simulink model "blockdiagram"  (R2020a)
settings: Solver=ode4  StartTime=0.0  StopTime=12  FixedStep=0.001  RelTol=1e-3
values from neighbouring files (symbols this model uses):
  B = 0.05    [ProblemA.m]
  J = 0.1    [ProblemA.m]
  L2 = (Lmax-Lmin)/2    (= 0.04)    [ProblemA.m]
  theta_m0 = 0    [ProblemA.m]
undefined symbols (not defined in the file or in its folder): sigbuilder_block
libraries: simulink x6
(part 2 of 2)

== system blockdiagram/If Action Subsystem3/If Action Subsystem3 ==
  In1 : Inport
  Action Port : ActionPort  InitializeStates=reset  ActionPortLabel=if(u1 <-ep)
  Out1 : Outport
  wires:
  In1/1 -> Out1/1

== system blockdiagram/If Action Subsystem4/If Action Subsystem1 ==
  In1 : Inport
  Action Port : ActionPort  ActionPortLabel=else
  Constant14 : Constant  Value=-2*pi
  Mod13 : Math  Operator=mod  SaturateOnIntegerOverflow=on
  Out1 : Outport
  wires:
  In1/1 -> Mod13/1
  Constant14/1 -> Mod13/2
  Mod13/1 -> Out1/1

== system blockdiagram/If Action Subsystem4/If Action Subsystem3 ==
  In1 : Inport
  Action Port : ActionPort  InitializeStates=reset  ActionPortLabel=if(u1 <-ep)
  Out1 : Outport
  wires:
  In1/1 -> Out1/1

== system blockdiagram/If Action Subsystem5/Subsystem7 ==
  In1 : Inport
  Derivative1 : Derivative
  If Action Subsystem1 : Subsystem  TreatAsAtomicUnit=on
  If Action Subsystem3 : Subsystem  TreatAsAtomicUnit=on
  If2 : If  IfExpression=u1 < 0
  Merge2 : Merge
  Out1 : Outport
  wires:
  Derivative1/1 -> If2/1
  If2/2 -> If Action Subsystem1/Action
  If Action Subsystem1/1(Out1) -> Merge2/2
  If Action Subsystem3/1(Out2) -> Merge2/1
  If2/1 -> If Action Subsystem3/Action
  In1/1 -> If Action Subsystem3/1(In2), If Action Subsystem1/1(In1), Derivative1/1
  Merge2/1 -> Out1/1

== system blockdiagram/If Action Subsystem7/If Action Subsystem1 ==
  In1 : Inport
  Action Port : ActionPort  ActionPortLabel=if(u1<1.772)
  Subsystem7 : Subsystem
  Out1 : Outport
  wires:
  In1/1 -> Subsystem7/1(In1)
  Subsystem7/1(Out1) -> Out1/1

== system blockdiagram/If Action Subsystem7/If Action Subsystem7 ==
  In1 : Inport
  Action Port : ActionPort  ActionPortLabel=else
  Clock1 : Clock
  If Action Subsystem1 : Subsystem  TreatAsAtomicUnit=on
  If Action Subsystem7 : Subsystem  TreatAsAtomicUnit=on
  If4 : If  IfExpression=u1>9.658
  Merge2 : Merge
  Subsystem7 : Subsystem
  Out1 : Outport
  wires:
  Merge2/1 -> Out1/1
  If Action Subsystem7/1(Out1) -> Merge2/2
  In1/1 -> If Action Subsystem7/1(In1), If Action Subsystem1/1(In1)
  If4/2 -> If Action Subsystem7/Action
  Clock1/1 -> If4/1
  If4/1 -> If Action Subsystem1/Action
  If Action Subsystem1/1(Out1) -> Merge2/1

== system blockdiagram/If Action Subsystem7/Subsystem7 ==
  In1 : Inport
  Derivative1 : Derivative
  If Action Subsystem1 : Subsystem  TreatAsAtomicUnit=on
  If Action Subsystem3 : Subsystem  TreatAsAtomicUnit=on
  If2 : If  IfExpression=u1 < 0
  Merge2 : Merge
  Out1 : Outport
  wires:
  Derivative1/1 -> If2/1
  If2/2 -> If Action Subsystem1/Action
  If Action Subsystem1/1(Out1) -> Merge2/2
  If Action Subsystem3/1(Out2) -> Merge2/1
  If2/1 -> If Action Subsystem3/Action
  In1/1 -> If Action Subsystem3/1(In2), If Action Subsystem1/1(In1), Derivative1/1
  Merge2/1 -> Out1/1

== system blockdiagram/Subsystem/If Action Subsystem1 ==
  In1 : Inport
  Action Port : ActionPort  ActionPortLabel=else
  If Action Subsystem2 : Subsystem  TreatAsAtomicUnit=on
  If Action Subsystem4 : Subsystem  TreatAsAtomicUnit=on
  If1 : If  IfExpression=u1 <ep
  Merge1 : Merge
  Out1 : Outport
  wires:
  If1/1 -> If Action Subsystem4/Action
  If1/2 -> If Action Subsystem2/Action
  Merge1/1 -> Out1/1
  If Action Subsystem4/1(Out1) -> Merge1/1
  If Action Subsystem2/1(Out1) -> Merge1/2
  In1/1 -> If Action Subsystem2/1(In1), If Action Subsystem4/1(In1), If1/1

== system blockdiagram/Subsystem/If Action Subsystem3 ==
  In2 : Inport
  Action Port : ActionPort  InitializeStates=reset  ActionPortLabel=if(u1 < 0)
  Add : Sum  Inputs=+-
  Constant : Constant  Value=2*pi
  Constant14 : Constant  Value=-2*pi
  If Action Subsystem1 : Subsystem  TreatAsAtomicUnit=on
  If Action Subsystem3 : Subsystem  TreatAsAtomicUnit=on
  If2 : If  IfExpression=u1 <-ep
  Merge2 : Merge
  Mod13 : Math  Operator=mod  SaturateOnIntegerOverflow=on
  Out2 : Outport
  wires:
  Mod13/1 -> ?
  Constant14/1 -> Mod13/2
  ? -> Mod13/1
  Constant/1 -> Add/2
  In2/1 -> If Action Subsystem1/1(In1), If Action Subsystem3/1(In1), If2/1
  If Action Subsystem3/1(Out1) -> Merge2/1
  If2/1 -> If Action Subsystem3/Action
  If Action Subsystem1/1(Out1) -> Merge2/2
  If2/2 -> If Action Subsystem1/Action
  Merge2/1 -> Out2/1

== system blockdiagram/Subsystem1/If Action Subsystem1 ==
  In1 : Inport
  Action Port : ActionPort  ActionPortLabel=else
  Constant14 : Constant  Value=2*pi
  Mod13 : Math  Operator=mod  SaturateOnIntegerOverflow=on
  Out1 : Outport
  wires:
  In1/1 -> Mod13/1
  Constant14/1 -> Mod13/2
  Mod13/1 -> Out1/1

== system blockdiagram/Subsystem1/If Action Subsystem3 ==
  In1 : Inport
  Action Port : ActionPort  InitializeStates=reset  ActionPortLabel=if(u1 <ep)
  Out1 : Outport
  wires:
  In1/1 -> Out1/1

== system blockdiagram/Subsystem2/If Action Subsystem1 ==
  In1 : Inport
  Action Port : ActionPort  ActionPortLabel=else
  Constant14 : Constant  Value=2*pi
  Mod13 : Math  Operator=mod  SaturateOnIntegerOverflow=on
  Out1 : Outport
  wires:
  In1/1 -> Mod13/1
  Constant14/1 -> Mod13/2
  Mod13/1 -> Out1/1

== system blockdiagram/Subsystem2/If Action Subsystem3 ==
  In1 : Inport
  Action Port : ActionPort  InitializeStates=reset  ActionPortLabel=if(u1 <ep)
  Out1 : Outport
  wires:
  In1/1 -> Out1/1

== system blockdiagram/Subsystem3/If Action Subsystem1 ==
  In1 : Inport
  Action Port : ActionPort  ActionPortLabel=else
  Constant14 : Constant  Value=-2*pi
  Mod13 : Math  Operator=mod  SaturateOnIntegerOverflow=on
  Out1 : Outport
  wires:
  In1/1 -> Mod13/1
  Constant14/1 -> Mod13/2
  Mod13/1 -> Out1/1

== system blockdiagram/Subsystem3/If Action Subsystem3 ==
  In1 : Inport
  Action Port : ActionPort  InitializeStates=reset  ActionPortLabel=if(u1 <-ep)
  Out1 : Outport
  wires:
  In1/1 -> Out1/1

== system blockdiagram/Subsystem4/If Action Subsystem1 ==
  In1 : Inport
  Action Port : ActionPort  ActionPortLabel=else
  Constant14 : Constant  Value=-2*pi
  Mod13 : Math  Operator=mod  SaturateOnIntegerOverflow=on
  Out1 : Outport
  wires:
  In1/1 -> Mod13/1
  Constant14/1 -> Mod13/2
  Mod13/1 -> Out1/1

== system blockdiagram/Subsystem4/If Action Subsystem3 ==
  In1 : Inport
  Action Port : ActionPort  InitializeStates=reset  ActionPortLabel=if(u1 >-ep)
  Out1 : Outport
  wires:
  In1/1 -> Out1/1

== system blockdiagram/Subsystem5/If Action Subsystem1 ==
  In1 : Inport
  Action Port : ActionPort  ActionPortLabel=else
  If Action Subsystem2 : Subsystem  TreatAsAtomicUnit=on
  If Action Subsystem4 : Subsystem  TreatAsAtomicUnit=on
  If1 : If  IfExpression=u1 <ep
  Merge1 : Merge
  Out1 : Outport
  wires:
  If1/1 -> If Action Subsystem4/Action
  If1/2 -> If Action Subsystem2/Action
  Merge1/1 -> Out1/1
  If Action Subsystem4/1(Out1) -> Merge1/1
  If Action Subsystem2/1(Out1) -> Merge1/2
  In1/1 -> If Action Subsystem2/1(In1), If Action Subsystem4/1(In1), If1/1

== system blockdiagram/Subsystem5/If Action Subsystem3 ==
  In2 : Inport
  Action Port : ActionPort  InitializeStates=reset  ActionPortLabel=if(u1 < 0)
  Add : Sum  Inputs=+-
  Constant : Constant  Value=2*pi
  Constant14 : Constant  Value=-2*pi
  If Action Subsystem1 : Subsystem  TreatAsAtomicUnit=on
  If Action Subsystem3 : Subsystem  TreatAsAtomicUnit=on
  If2 : If  IfExpression=u1 <-ep
  Merge2 : Merge
  Mod13 : Math  Operator=mod  SaturateOnIntegerOverflow=on
  Out2 : Outport
  wires:
  Mod13/1 -> ?
  Constant14/1 -> Mod13/2
  ? -> Mod13/1
  Constant/1 -> Add/2
  In2/1 -> If Action Subsystem1/1(In1), If Action Subsystem3/1(In1), If2/1
  If Action Subsystem3/1(Out1) -> Merge2/1
  If2/1 -> If Action Subsystem3/Action
  If Action Subsystem1/1(Out1) -> Merge2/2
  If2/2 -> If Action Subsystem1/Action
  Merge2/1 -> Out2/1

== system blockdiagram/Subsystem6/If Action Subsystem1 ==
  In1 : Inport
  Action Port : ActionPort  ActionPortLabel=else
  If Action Subsystem2 : Subsystem  TreatAsAtomicUnit=on
  If Action Subsystem4 : Subsystem  TreatAsAtomicUnit=on
  If1 : If  IfExpression=u1 <ep
  Merge1 : Merge
  Out1 : Outport
  wires:
  If1/1 -> If Action Subsystem4/Action
  If1/2 -> If Action Subsystem2/Action
  Merge1/1 -> Out1/1
  If Action Subsystem4/1(Out1) -> Merge1/1
  If Action Subsystem2/1(Out1) -> Merge1/2
  In1/1 -> If Action Subsystem2/1(In1), If Action Subsystem4/1(In1), If1/1

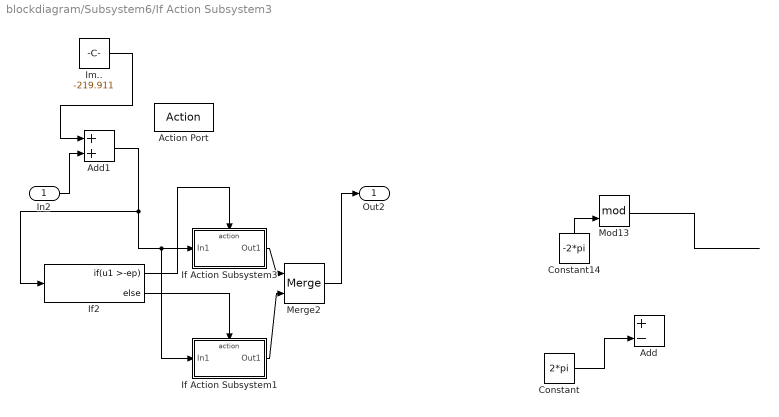
== system blockdiagram/Subsystem6/If Action Subsystem3 ==
  In2 : Inport
  Action Port : ActionPort  InitializeStates=reset  ActionPortLabel=if(u1 < 0)
  Add : Sum  Inputs=+-
  Add1 : Sum
  Constant : Constant  Value=2*pi
  Constant14 : Constant  Value=-2*pi
  If Action Subsystem1 : Subsystem  TreatAsAtomicUnit=on
  If Action Subsystem3 : Subsystem  TreatAsAtomicUnit=on
  If2 : If  IfExpression=u1 >-ep
  Im.. : Constant  Value=-219.911
  Merge2 : Merge
  Mod13 : Math  Operator=mod  SaturateOnIntegerOverflow=on
  Out2 : Outport
  wires:
  Mod13/1 -> ?
  Constant14/1 -> Mod13/2
  ? -> Mod13/1
  Constant/1 -> Add/2
  If Action Subsystem3/1(Out1) -> Merge2/1
  If2/1 -> If Action Subsystem3/Action
  If Action Subsystem1/1(Out1) -> Merge2/2
  If2/2 -> If Action Subsystem1/Action
  Merge2/1 -> Out2/1
  Im../1 -> Add1/1
  In2/1 -> Add1/2
  Add1/1 -> If Action Subsystem3/1(In1), If Action Subsystem1/1(In1), If2/1

== system blockdiagram/Subsystem7/If Action Subsystem1 ==
  In1 : Inport
  Action Port : ActionPort  ActionPortLabel=else
  If Action Subsystem2 : Subsystem  TreatAsAtomicUnit=on
  If Action Subsystem4 : Subsystem  TreatAsAtomicUnit=on
  If1 : If  IfExpression=u1 <ep
  Merge1 : Merge
  Out1 : Outport
  wires:
  If1/1 -> If Action Subsystem4/Action
  If1/2 -> If Action Subsystem2/Action
  Merge1/1 -> Out1/1
  If Action Subsystem4/1(Out1) -> Merge1/1
  If Action Subsystem2/1(Out1) -> Merge1/2
  In1/1 -> If Action Subsystem2/1(In1), If Action Subsystem4/1(In1), If1/1

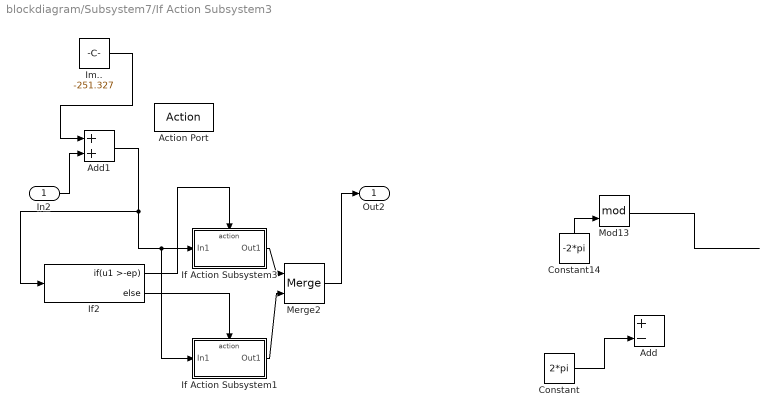
== system blockdiagram/Subsystem7/If Action Subsystem3 ==
  In2 : Inport
  Action Port : ActionPort  InitializeStates=reset  ActionPortLabel=if(u1 < 0)
  Add : Sum  Inputs=+-
  Add1 : Sum
  Constant : Constant  Value=2*pi
  Constant14 : Constant  Value=-2*pi
  If Action Subsystem1 : Subsystem  TreatAsAtomicUnit=on
  If Action Subsystem3 : Subsystem  TreatAsAtomicUnit=on
  If2 : If  IfExpression=u1 >-ep
  Im.. : Constant  Value=-251.327
  Merge2 : Merge
  Mod13 : Math  Operator=mod  SaturateOnIntegerOverflow=on
  Out2 : Outport
  wires:
  Mod13/1 -> ?
  Constant14/1 -> Mod13/2
  ? -> Mod13/1
  Constant/1 -> Add/2
  If Action Subsystem3/1(Out1) -> Merge2/1
  If2/1 -> If Action Subsystem3/Action
  If Action Subsystem1/1(Out1) -> Merge2/2
  If2/2 -> If Action Subsystem1/Action
  Merge2/1 -> Out2/1
  Im../1 -> Add1/1
  In2/1 -> Add1/2
  Add1/1 -> If Action Subsystem3/1(In1), If Action Subsystem1/1(In1), If2/1

== system blockdiagram/Subsystem8/If Action Subsystem1 ==
  In1 : Inport
  Action Port : ActionPort  ActionPortLabel=else
  If Action Subsystem2 : Subsystem  TreatAsAtomicUnit=on
  If Action Subsystem4 : Subsystem  TreatAsAtomicUnit=on
  If1 : If  IfExpression=u1 <ep
  Merge1 : Merge
  Out1 : Outport
  wires:
  If1/1 -> If Action Subsystem4/Action
  If1/2 -> If Action Subsystem2/Action
  Merge1/1 -> Out1/1
  If Action Subsystem4/1(Out1) -> Merge1/1
  If Action Subsystem2/1(Out1) -> Merge1/2
  In1/1 -> If Action Subsystem2/1(In1), If Action Subsystem4/1(In1), If1/1

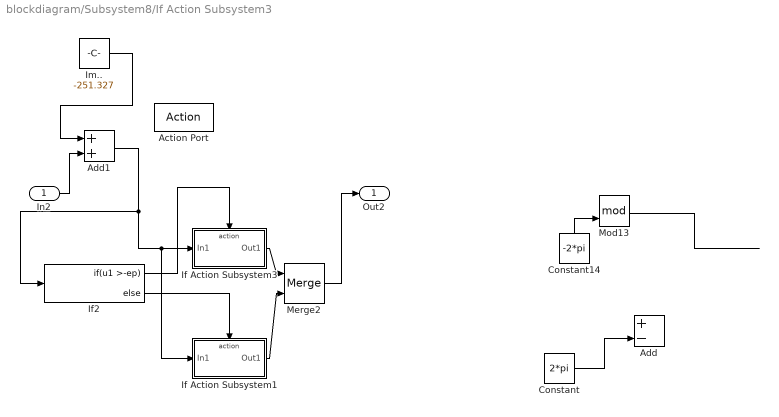
== system blockdiagram/Subsystem8/If Action Subsystem3 ==
  In2 : Inport
  Action Port : ActionPort  InitializeStates=reset  ActionPortLabel=if(u1 < 0)
  Add : Sum  Inputs=+-
  Add1 : Sum
  Constant : Constant  Value=2*pi
  Constant14 : Constant  Value=-2*pi
  If Action Subsystem1 : Subsystem  TreatAsAtomicUnit=on
  If Action Subsystem3 : Subsystem  TreatAsAtomicUnit=on
  If2 : If  IfExpression=u1 >-ep
  Im.. : Constant  Value=-251.327
  Merge2 : Merge
  Mod13 : Math  Operator=mod  SaturateOnIntegerOverflow=on
  Out2 : Outport
  wires:
  Mod13/1 -> ?
  Constant14/1 -> Mod13/2
  ? -> Mod13/1
  Constant/1 -> Add/2
  If Action Subsystem3/1(Out1) -> Merge2/1
  If2/1 -> If Action Subsystem3/Action
  If Action Subsystem1/1(Out1) -> Merge2/2
  If2/2 -> If Action Subsystem1/Action
  Merge2/1 -> Out2/1
  Im../1 -> Add1/1
  In2/1 -> Add1/2
  Add1/1 -> If Action Subsystem3/1(In1), If Action Subsystem1/1(In1), If2/1

== system blockdiagram/If Action Subsystem5/Subsystem7/If Action Subsystem1 ==
  In1 : Inport
  Action Port : ActionPort  ActionPortLabel=else
  If Action Subsystem2 : Subsystem  TreatAsAtomicUnit=on
  If Action Subsystem4 : Subsystem  TreatAsAtomicUnit=on
  If1 : If  IfExpression=u1 <ep
  Merge1 : Merge
  Out1 : Outport
  wires:
  If1/1 -> If Action Subsystem4/Action
  If1/2 -> If Action Subsystem2/Action
  Merge1/1 -> Out1/1
  If Action Subsystem4/1(Out1) -> Merge1/1
  If Action Subsystem2/1(Out1) -> Merge1/2
  In1/1 -> If Action Subsystem2/1(In1), If Action Subsystem4/1(In1), If1/1

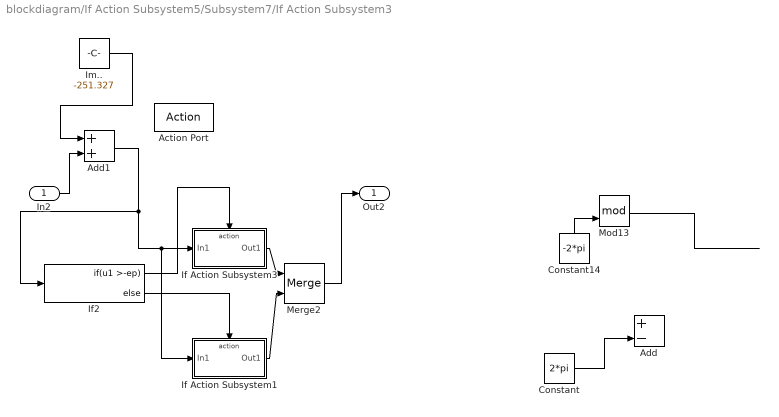
== system blockdiagram/If Action Subsystem5/Subsystem7/If Action Subsystem3 ==
  In2 : Inport
  Action Port : ActionPort  InitializeStates=reset  ActionPortLabel=if(u1 < 0)
  Add : Sum  Inputs=+-
  Add1 : Sum
  Constant : Constant  Value=2*pi
  Constant14 : Constant  Value=-2*pi
  If Action Subsystem1 : Subsystem  TreatAsAtomicUnit=on
  If Action Subsystem3 : Subsystem  TreatAsAtomicUnit=on
  If2 : If  IfExpression=u1 >-ep
  Im.. : Constant  Value=-251.327
  Merge2 : Merge
  Mod13 : Math  Operator=mod  SaturateOnIntegerOverflow=on
  Out2 : Outport
  wires:
  Mod13/1 -> ?
  Constant14/1 -> Mod13/2
  ? -> Mod13/1
  Constant/1 -> Add/2
  If Action Subsystem3/1(Out1) -> Merge2/1
  If2/1 -> If Action Subsystem3/Action
  If Action Subsystem1/1(Out1) -> Merge2/2
  If2/2 -> If Action Subsystem1/Action
  Merge2/1 -> Out2/1
  Im../1 -> Add1/1
  In2/1 -> Add1/2
  Add1/1 -> If Action Subsystem3/1(In1), If Action Subsystem1/1(In1), If2/1

== system blockdiagram/If Action Subsystem7/If Action Subsystem1/Subsystem7 ==
  In1 : Inport
  Derivative1 : Derivative
  If Action Subsystem1 : Subsystem  TreatAsAtomicUnit=on
  If Action Subsystem3 : Subsystem  TreatAsAtomicUnit=on
  If2 : If  IfExpression=u1 < 0
  Merge2 : Merge
  Out1 : Outport
  wires:
  Derivative1/1 -> If2/1
  If2/2 -> If Action Subsystem1/Action
  If Action Subsystem1/1(Out1) -> Merge2/2
  If Action Subsystem3/1(Out2) -> Merge2/1
  If2/1 -> If Action Subsystem3/Action
  In1/1 -> If Action Subsystem3/1(In2), If Action Subsystem1/1(In1), Derivative1/1
  Merge2/1 -> Out1/1

== system blockdiagram/If Action Subsystem7/If Action Subsystem7/If Action Subsystem1 ==
  In1 : Inport
  Action Port : ActionPort  ActionPortLabel=if(u1>9.658)
  Subsystem7 : Subsystem
  Out1 : Outport
  wires:
  In1/1 -> Subsystem7/1(In1)
  Subsystem7/1(Out1) -> Out1/1

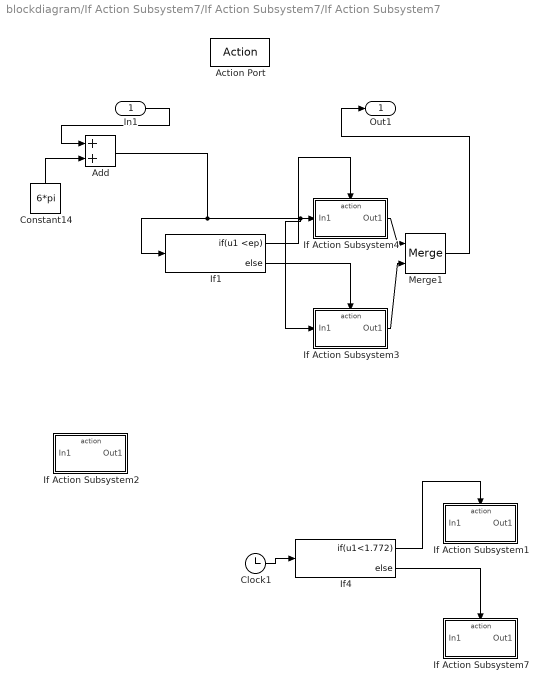
== system blockdiagram/If Action Subsystem7/If Action Subsystem7/If Action Subsystem7 ==
  In1 : Inport
  Action Port : ActionPort  ActionPortLabel=else
  Add : Sum
  Clock1 : Clock
  Constant14 : Constant  Value=6*pi
  If Action Subsystem1 : Subsystem  TreatAsAtomicUnit=on
  If Action Subsystem2 : Subsystem  TreatAsAtomicUnit=on
  If Action Subsystem3 : Subsystem  TreatAsAtomicUnit=on
  If Action Subsystem4 : Subsystem  TreatAsAtomicUnit=on
  If Action Subsystem7 : Subsystem  TreatAsAtomicUnit=on
  If1 : If  IfExpression=u1 <ep
  If4 : If  IfExpression=u1<1.772
  Merge1 : Merge
  Out1 : Outport
  wires:
  Merge1/1 -> Out1/1
  If4/2 -> If Action Subsystem7/Action
  Clock1/1 -> If4/1
  ? -> If Action Subsystem1/1(In1), If Action Subsystem7/1(In1)
  If4/1 -> If Action Subsystem1/Action
  If1/1 -> If Action Subsystem4/Action
  If Action Subsystem4/1(Out1) -> Merge1/1
  If1/2 -> If Action Subsystem3/Action
  If Action Subsystem3/1(Out1) -> Merge1/2
  Add/1 -> If1/1, If Action Subsystem3/1(In1), If Action Subsystem4/1(In1)
  In1/1 -> Add/1
  Constant14/1 -> Add/2

== system blockdiagram/If Action Subsystem7/If Action Subsystem7/Subsystem7 ==
  In1 : Inport
  Derivative1 : Derivative
  If Action Subsystem1 : Subsystem  TreatAsAtomicUnit=on
  If Action Subsystem3 : Subsystem  TreatAsAtomicUnit=on
  If2 : If  IfExpression=u1 < 0
  Merge2 : Merge
  Out1 : Outport
  wires:
  Derivative1/1 -> If2/1
  If2/2 -> If Action Subsystem1/Action
  If Action Subsystem1/1(Out1) -> Merge2/2
  If Action Subsystem3/1(Out2) -> Merge2/1
  If2/1 -> If Action Subsystem3/Action
  In1/1 -> If Action Subsystem3/1(In2), If Action Subsystem1/1(In1), Derivative1/1
  Merge2/1 -> Out1/1

== system blockdiagram/If Action Subsystem7/Subsystem7/If Action Subsystem1 ==
  In1 : Inport
  Action Port : ActionPort  ActionPortLabel=else
  If Action Subsystem2 : Subsystem  TreatAsAtomicUnit=on
  If Action Subsystem4 : Subsystem  TreatAsAtomicUnit=on
  If1 : If  IfExpression=u1 <ep
  Merge1 : Merge
  Out1 : Outport
  wires:
  If1/1 -> If Action Subsystem4/Action
  If1/2 -> If Action Subsystem2/Action
  Merge1/1 -> Out1/1
  If Action Subsystem4/1(Out1) -> Merge1/1
  If Action Subsystem2/1(Out1) -> Merge1/2
  In1/1 -> If Action Subsystem2/1(In1), If Action Subsystem4/1(In1), If1/1

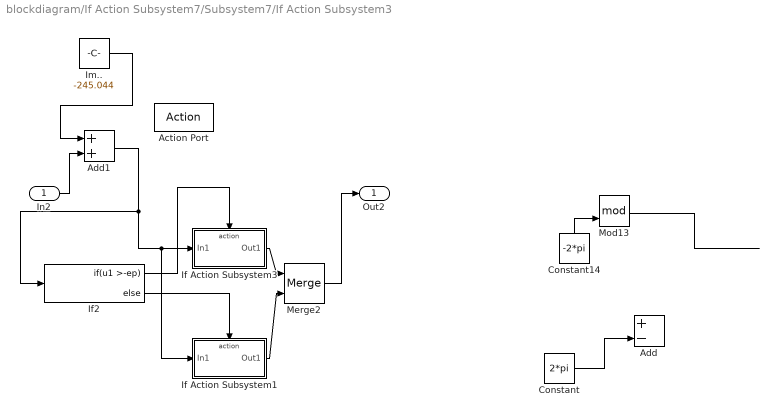
== system blockdiagram/If Action Subsystem7/Subsystem7/If Action Subsystem3 ==
  In2 : Inport
  Action Port : ActionPort  InitializeStates=reset  ActionPortLabel=if(u1 < 0)
  Add : Sum  Inputs=+-
  Add1 : Sum
  Constant : Constant  Value=2*pi
  Constant14 : Constant  Value=-2*pi
  If Action Subsystem1 : Subsystem  TreatAsAtomicUnit=on
  If Action Subsystem3 : Subsystem  TreatAsAtomicUnit=on
  If2 : If  IfExpression=u1 >-ep
  Im.. : Constant  Value=-245.044
  Merge2 : Merge
  Mod13 : Math  Operator=mod  SaturateOnIntegerOverflow=on
  Out2 : Outport
  wires:
  Mod13/1 -> ?
  Constant14/1 -> Mod13/2
  ? -> Mod13/1
  Constant/1 -> Add/2
  If Action Subsystem3/1(Out1) -> Merge2/1
  If2/1 -> If Action Subsystem3/Action
  If Action Subsystem1/1(Out1) -> Merge2/2
  If2/2 -> If Action Subsystem1/Action
  Merge2/1 -> Out2/1
  Im../1 -> Add1/1
  In2/1 -> Add1/2
  Add1/1 -> If Action Subsystem3/1(In1), If Action Subsystem1/1(In1), If2/1

== system blockdiagram/Subsystem/If Action Subsystem1/If Action Subsystem2 ==
  In1 : Inport
  Action Port : ActionPort  ActionPortLabel=else
  Constant14 : Constant  Value=2*pi
  Mod13 : Math  Operator=mod  SaturateOnIntegerOverflow=on
  Out1 : Outport
  wires:
  In1/1 -> Mod13/1
  Constant14/1 -> Mod13/2
  Mod13/1 -> Out1/1

== system blockdiagram/Subsystem/If Action Subsystem1/If Action Subsystem4 ==
  In1 : Inport
  Action Port : ActionPort  InitializeStates=reset  ActionPortLabel=if(u1 <ep)
  Out1 : Outport
  wires:
  In1/1 -> Out1/1

== system blockdiagram/Subsystem/If Action Subsystem3/If Action Subsystem1 ==
  In1 : Inport
  Action Port : ActionPort  ActionPortLabel=else
  Constant14 : Constant  Value=-2*pi
  Mod13 : Math  Operator=mod  SaturateOnIntegerOverflow=on
  Out1 : Outport
  wires:
  In1/1 -> Mod13/1
  Constant14/1 -> Mod13/2
  Mod13/1 -> Out1/1

== system blockdiagram/Subsystem/If Action Subsystem3/If Action Subsystem3 ==
  In1 : Inport
  Action Port : ActionPort  InitializeStates=reset  ActionPortLabel=if(u1 <-ep)
  Out1 : Outport
  wires:
  In1/1 -> Out1/1

== system blockdiagram/Subsystem5/If Action Subsystem1/If Action Subsystem2 ==
  In1 : Inport
  Action Port : ActionPort  ActionPortLabel=else
  Constant14 : Constant  Value=2*pi
  Mod13 : Math  Operator=mod  SaturateOnIntegerOverflow=on
  Out1 : Outport
  wires:
  In1/1 -> Mod13/1
  Constant14/1 -> Mod13/2
  Mod13/1 -> Out1/1

== system blockdiagram/Subsystem5/If Action Subsystem1/If Action Subsystem4 ==
  In1 : Inport
  Action Port : ActionPort  InitializeStates=reset  ActionPortLabel=if(u1 <ep)
  Out1 : Outport
  wires:
  In1/1 -> Out1/1

== system blockdiagram/Subsystem5/If Action Subsystem3/If Action Subsystem1 ==
  In1 : Inport
  Action Port : ActionPort  ActionPortLabel=else
  Constant14 : Constant  Value=-2*pi
  Mod13 : Math  Operator=mod  SaturateOnIntegerOverflow=on
  Out1 : Outport
  wires:
  In1/1 -> Mod13/1
  Constant14/1 -> Mod13/2
  Mod13/1 -> Out1/1

== system blockdiagram/Subsystem5/If Action Subsystem3/If Action Subsystem3 ==
  In1 : Inport
  Action Port : ActionPort  InitializeStates=reset  ActionPortLabel=if(u1 <-ep)
  Out1 : Outport
  wires:
  In1/1 -> Out1/1

== system blockdiagram/Subsystem6/If Action Subsystem1/If Action Subsystem2 ==
  In1 : Inport
  Action Port : ActionPort  ActionPortLabel=else
  Constant14 : Constant  Value=2*pi
  Mod13 : Math  Operator=mod  SaturateOnIntegerOverflow=on
  Out1 : Outport
  wires:
  In1/1 -> Mod13/1
  Constant14/1 -> Mod13/2
  Mod13/1 -> Out1/1

== system blockdiagram/Subsystem6/If Action Subsystem1/If Action Subsystem4 ==
  In1 : Inport
  Action Port : ActionPort  InitializeStates=reset  ActionPortLabel=if(u1 <ep)
  Out1 : Outport
  wires:
  In1/1 -> Out1/1

== system blockdiagram/Subsystem6/If Action Subsystem3/If Action Subsystem1 ==
  In1 : Inport
  Action Port : ActionPort  ActionPortLabel=else
  Constant14 : Constant  Value=-2*pi
  Mod13 : Math  Operator=mod  SaturateOnIntegerOverflow=on
  Out1 : Outport
  wires:
  In1/1 -> Mod13/1
  Constant14/1 -> Mod13/2
  Mod13/1 -> Out1/1

== system blockdiagram/Subsystem6/If Action Subsystem3/If Action Subsystem3 ==
  In1 : Inport
  Action Port : ActionPort  InitializeStates=reset  ActionPortLabel=if(u1 >-ep)
  Out1 : Outport
  wires:
  In1/1 -> Out1/1

== system blockdiagram/Subsystem7/If Action Subsystem1/If Action Subsystem2 ==
  In1 : Inport
  Action Port : ActionPort  ActionPortLabel=else
  Constant14 : Constant  Value=2*pi
  Mod13 : Math  Operator=mod  SaturateOnIntegerOverflow=on
  Out1 : Outport
  wires:
  In1/1 -> Mod13/1
  Constant14/1 -> Mod13/2
  Mod13/1 -> Out1/1

== system blockdiagram/Subsystem7/If Action Subsystem1/If Action Subsystem4 ==
  In1 : Inport
  Action Port : ActionPort  InitializeStates=reset  ActionPortLabel=if(u1 <ep)
  Out1 : Outport
  wires:
  In1/1 -> Out1/1

== system blockdiagram/Subsystem7/If Action Subsystem3/If Action Subsystem1 ==
  In1 : Inport
  Action Port : ActionPort  ActionPortLabel=else
  Constant14 : Constant  Value=-2*pi
  Mod13 : Math  Operator=mod  SaturateOnIntegerOverflow=on
  Out1 : Outport
  wires:
  In1/1 -> Mod13/1
  Constant14/1 -> Mod13/2
  Mod13/1 -> Out1/1

== system blockdiagram/Subsystem7/If Action Subsystem3/If Action Subsystem3 ==
  In1 : Inport
  Action Port : ActionPort  InitializeStates=reset  ActionPortLabel=if(u1 >-ep)
  Out1 : Outport
  wires:
  In1/1 -> Out1/1

== system blockdiagram/Subsystem8/If Action Subsystem1/If Action Subsystem2 ==
  In1 : Inport
  Action Port : ActionPort  ActionPortLabel=else
  Constant14 : Constant  Value=2*pi
  Mod13 : Math  Operator=mod  SaturateOnIntegerOverflow=on
  Out1 : Outport
  wires:
  In1/1 -> Mod13/1
  Constant14/1 -> Mod13/2
  Mod13/1 -> Out1/1

== system blockdiagram/Subsystem8/If Action Subsystem1/If Action Subsystem4 ==
  In1 : Inport
  Action Port : ActionPort  InitializeStates=reset  ActionPortLabel=if(u1 <ep)
  Out1 : Outport
  wires:
  In1/1 -> Out1/1

== system blockdiagram/Subsystem8/If Action Subsystem3/If Action Subsystem1 ==
  In1 : Inport
  Action Port : ActionPort  ActionPortLabel=else
  Constant14 : Constant  Value=-2*pi
  Mod13 : Math  Operator=mod  SaturateOnIntegerOverflow=on
  Out1 : Outport
  wires:
  In1/1 -> Mod13/1
  Constant14/1 -> Mod13/2
  Mod13/1 -> Out1/1

== system blockdiagram/Subsystem8/If Action Subsystem3/If Action Subsystem3 ==
  In1 : Inport
  Action Port : ActionPort  InitializeStates=reset  ActionPortLabel=if(u1 >-ep)
  Out1 : Outport
  wires:
  In1/1 -> Out1/1

== system blockdiagram/If Action Subsystem5/Subsystem7/If Action Subsystem1/If Action Subsystem2 ==
  In1 : Inport
  Action Port : ActionPort  ActionPortLabel=else
  Constant14 : Constant  Value=2*pi
  Mod13 : Math  Operator=mod  SaturateOnIntegerOverflow=on
  Out1 : Outport
  wires:
  In1/1 -> Mod13/1
  Constant14/1 -> Mod13/2
  Mod13/1 -> Out1/1

== system blockdiagram/If Action Subsystem5/Subsystem7/If Action Subsystem1/If Action Subsystem4 ==
  In1 : Inport
  Action Port : ActionPort  InitializeStates=reset  ActionPortLabel=if(u1 <ep)
  Out1 : Outport
  wires:
  In1/1 -> Out1/1

== system blockdiagram/If Action Subsystem5/Subsystem7/If Action Subsystem3/If Action Subsystem1 ==
  In1 : Inport
  Action Port : ActionPort  ActionPortLabel=else
  Constant14 : Constant  Value=-2*pi
  Mod13 : Math  Operator=mod  SaturateOnIntegerOverflow=on
  Out1 : Outport
  wires:
  In1/1 -> Mod13/1
  Constant14/1 -> Mod13/2
  Mod13/1 -> Out1/1

== system blockdiagram/If Action Subsystem5/Subsystem7/If Action Subsystem3/If Action Subsystem3 ==
  In1 : Inport
  Action Port : ActionPort  InitializeStates=reset  ActionPortLabel=if(u1 >-ep)
  Out1 : Outport
  wires:
  In1/1 -> Out1/1

== system blockdiagram/If Action Subsystem7/If Action Subsystem1/Subsystem7/If Action Subsystem1 ==
  In1 : Inport
  Action Port : ActionPort  ActionPortLabel=else
  If Action Subsystem2 : Subsystem  TreatAsAtomicUnit=on
  If Action Subsystem4 : Subsystem  TreatAsAtomicUnit=on
  If1 : If  IfExpression=u1 <ep
  Merge1 : Merge
  Out1 : Outport
  wires:
  If1/1 -> If Action Subsystem4/Action
  If1/2 -> If Action Subsystem2/Action
  Merge1/1 -> Out1/1
  If Action Subsystem4/1(Out1) -> Merge1/1
  If Action Subsystem2/1(Out1) -> Merge1/2
  In1/1 -> If Action Subsystem2/1(In1), If Action Subsystem4/1(In1), If1/1

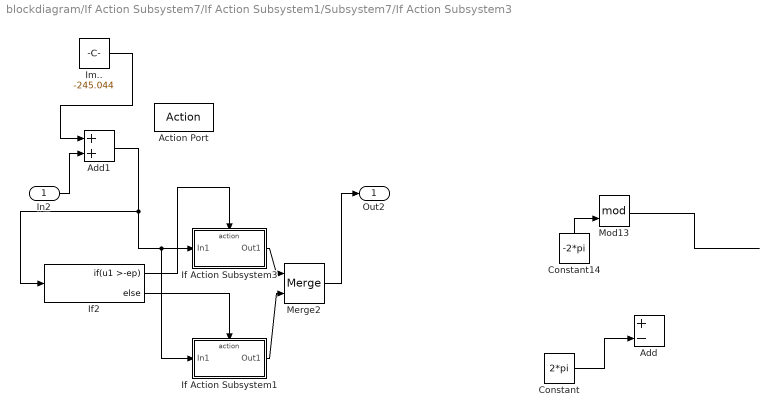
== system blockdiagram/If Action Subsystem7/If Action Subsystem1/Subsystem7/If Action Subsystem3 ==
  In2 : Inport
  Action Port : ActionPort  InitializeStates=reset  ActionPortLabel=if(u1 < 0)
  Add : Sum  Inputs=+-
  Add1 : Sum
  Constant : Constant  Value=2*pi
  Constant14 : Constant  Value=-2*pi
  If Action Subsystem1 : Subsystem  TreatAsAtomicUnit=on
  If Action Subsystem3 : Subsystem  TreatAsAtomicUnit=on
  If2 : If  IfExpression=u1 >-ep
  Im.. : Constant  Value=-245.044
  Merge2 : Merge
  Mod13 : Math  Operator=mod  SaturateOnIntegerOverflow=on
  Out2 : Outport
  wires:
  Mod13/1 -> ?
  Constant14/1 -> Mod13/2
  ? -> Mod13/1
  Constant/1 -> Add/2
  If Action Subsystem3/1(Out1) -> Merge2/1
  If2/1 -> If Action Subsystem3/Action
  If Action Subsystem1/1(Out1) -> Merge2/2
  If2/2 -> If Action Subsystem1/Action
  Merge2/1 -> Out2/1
  Im../1 -> Add1/1
  In2/1 -> Add1/2
  Add1/1 -> If Action Subsystem3/1(In1), If Action Subsystem1/1(In1), If2/1

== system blockdiagram/If Action Subsystem7/If Action Subsystem7/If Action Subsystem1/Subsystem7 ==
  In1 : Inport
  Derivative1 : Derivative
  If Action Subsystem1 : Subsystem  TreatAsAtomicUnit=on
  If Action Subsystem3 : Subsystem  TreatAsAtomicUnit=on
  If2 : If  IfExpression=u1 < 0
  Merge2 : Merge
  Out1 : Outport
  wires:
  Derivative1/1 -> If2/1
  If2/2 -> If Action Subsystem1/Action
  If Action Subsystem1/1(Out1) -> Merge2/2
  If Action Subsystem3/1(Out2) -> Merge2/1
  If2/1 -> If Action Subsystem3/Action
  In1/1 -> If Action Subsystem3/1(In2), If Action Subsystem1/1(In1), Derivative1/1
  Merge2/1 -> Out1/1

== system blockdiagram/If Action Subsystem7/If Action Subsystem7/If Action Subsystem7/If Action Subsystem1 ==
  In1 : Inport
  Action Port : ActionPort  ActionPortLabel=if(u1<1.772)
  Subsystem7 : Subsystem
  Out1 : Outport
  wires:
  In1/1 -> Subsystem7/1(In1)
  Subsystem7/1(Out1) -> Out1/1

== system blockdiagram/If Action Subsystem7/If Action Subsystem7/If Action Subsystem7/If Action Subsystem2 ==
  In1 : Inport
  Action Port : ActionPort
  If Action Subsystem2 : Subsystem  TreatAsAtomicUnit=on
  If Action Subsystem4 : Subsystem  TreatAsAtomicUnit=on
  If1 : If  IfExpression=u1 <ep
  Merge1 : Merge
  Out1 : Outport
  wires:
  If1/1 -> If Action Subsystem4/Action
  If1/2 -> If Action Subsystem2/Action
  Merge1/1 -> Out1/1
  If Action Subsystem4/1(Out1) -> Merge1/1
  If Action Subsystem2/1(Out1) -> Merge1/2
  In1/1 -> If Action Subsystem2/1(In1), If Action Subsystem4/1(In1), If1/1

== system blockdiagram/If Action Subsystem7/If Action Subsystem7/If Action Subsystem7/If Action Subsystem3 ==
  In1 : Inport
  Action Port : ActionPort  ActionPortLabel=else
  Constant14 : Constant  Value=2*pi
  Mod13 : Math  Operator=mod  SaturateOnIntegerOverflow=on
  Out1 : Outport
  wires:
  In1/1 -> Mod13/1
  Constant14/1 -> Mod13/2
  Mod13/1 -> Out1/1

== system blockdiagram/If Action Subsystem7/If Action Subsystem7/If Action Subsystem7/If Action Subsystem4 ==
  In1 : Inport
  Action Port : ActionPort  InitializeStates=reset  ActionPortLabel=if(u1 <ep)
  Out1 : Outport
  wires:
  In1/1 -> Out1/1

== system blockdiagram/If Action Subsystem7/If Action Subsystem7/If Action Subsystem7/If Action Subsystem7 ==
  In1 : Inport
  Action Port : ActionPort  ActionPortLabel=else
  Subsystem7 : Subsystem
  Out1 : Outport
  wires:
  In1/1 -> Subsystem7/1(In1)
  Subsystem7/1(Out1) -> Out1/1

== system blockdiagram/If Action Subsystem7/If Action Subsystem7/Subsystem7/If Action Subsystem1 ==
  In1 : Inport
  Action Port : ActionPort  ActionPortLabel=else
  If Action Subsystem2 : Subsystem  TreatAsAtomicUnit=on
  If Action Subsystem4 : Subsystem  TreatAsAtomicUnit=on
  If1 : If  IfExpression=u1 <ep
  Merge1 : Merge
  Out1 : Outport
  wires:
  If1/1 -> If Action Subsystem4/Action
  If1/2 -> If Action Subsystem2/Action
  Merge1/1 -> Out1/1
  If Action Subsystem4/1(Out1) -> Merge1/1
  If Action Subsystem2/1(Out1) -> Merge1/2
  In1/1 -> If Action Subsystem2/1(In1), If Action Subsystem4/1(In1), If1/1

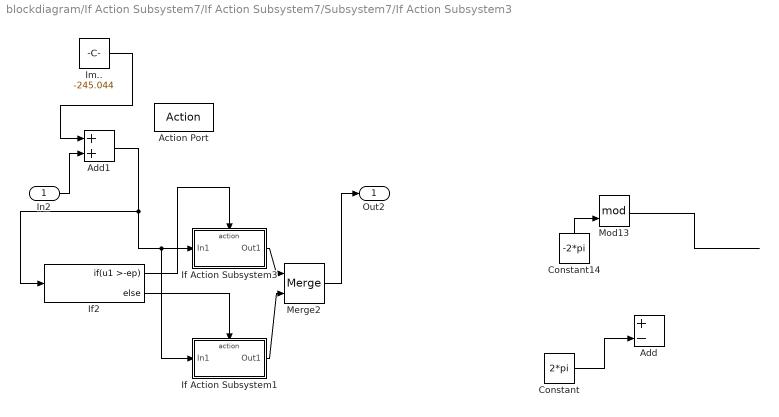
== system blockdiagram/If Action Subsystem7/If Action Subsystem7/Subsystem7/If Action Subsystem3 ==
  In2 : Inport
  Action Port : ActionPort  InitializeStates=reset  ActionPortLabel=if(u1 < 0)
  Add : Sum  Inputs=+-
  Add1 : Sum
  Constant : Constant  Value=2*pi
  Constant14 : Constant  Value=-2*pi
  If Action Subsystem1 : Subsystem  TreatAsAtomicUnit=on
  If Action Subsystem3 : Subsystem  TreatAsAtomicUnit=on
  If2 : If  IfExpression=u1 >-ep
  Im.. : Constant  Value=-245.044
  Merge2 : Merge
  Mod13 : Math  Operator=mod  SaturateOnIntegerOverflow=on
  Out2 : Outport
  wires:
  Mod13/1 -> ?
  Constant14/1 -> Mod13/2
  ? -> Mod13/1
  Constant/1 -> Add/2
  If Action Subsystem3/1(Out1) -> Merge2/1
  If2/1 -> If Action Subsystem3/Action
  If Action Subsystem1/1(Out1) -> Merge2/2
  If2/2 -> If Action Subsystem1/Action
  Merge2/1 -> Out2/1
  Im../1 -> Add1/1
  In2/1 -> Add1/2
  Add1/1 -> If Action Subsystem3/1(In1), If Action Subsystem1/1(In1), If2/1

== system blockdiagram/If Action Subsystem7/Subsystem7/If Action Subsystem1/If Action Subsystem2 ==
  In1 : Inport
  Action Port : ActionPort  ActionPortLabel=else
  Constant14 : Constant  Value=2*pi
  Mod13 : Math  Operator=mod  SaturateOnIntegerOverflow=on
  Out1 : Outport
  wires:
  In1/1 -> Mod13/1
  Constant14/1 -> Mod13/2
  Mod13/1 -> Out1/1

== system blockdiagram/If Action Subsystem7/Subsystem7/If Action Subsystem1/If Action Subsystem4 ==
  In1 : Inport
  Action Port : ActionPort  InitializeStates=reset  ActionPortLabel=if(u1 <ep)
  Out1 : Outport
  wires:
  In1/1 -> Out1/1

== system blockdiagram/If Action Subsystem7/Subsystem7/If Action Subsystem3/If Action Subsystem1 ==
  In1 : Inport
  Action Port : ActionPort  ActionPortLabel=else
  Constant14 : Constant  Value=-2*pi
  Mod13 : Math  Operator=mod  SaturateOnIntegerOverflow=on
  Out1 : Outport
  wires:
  In1/1 -> Mod13/1
  Constant14/1 -> Mod13/2
  Mod13/1 -> Out1/1

== system blockdiagram/If Action Subsystem7/Subsystem7/If Action Subsystem3/If Action Subsystem3 ==
  In1 : Inport
  Action Port : ActionPort  InitializeStates=reset  ActionPortLabel=if(u1 >-ep)
  Out1 : Outport
  wires:
  In1/1 -> Out1/1

== system blockdiagram/If Action Subsystem7/If Action Subsystem1/Subsystem7/If Action Subsystem1/If Action Subsystem2 ==
  In1 : Inport
  Action Port : ActionPort  ActionPortLabel=else
  Constant14 : Constant  Value=2*pi
  Mod13 : Math  Operator=mod  SaturateOnIntegerOverflow=on
  Out1 : Outport
  wires:
  In1/1 -> Mod13/1
  Constant14/1 -> Mod13/2
  Mod13/1 -> Out1/1

== system blockdiagram/If Action Subsystem7/If Action Subsystem1/Subsystem7/If Action Subsystem1/If Action Subsystem4 ==
  In1 : Inport
  Action Port : ActionPort  InitializeStates=reset  ActionPortLabel=if(u1 <ep)
  Out1 : Outport
  wires:
  In1/1 -> Out1/1

== system blockdiagram/If Action Subsystem7/If Action Subsystem1/Subsystem7/If Action Subsystem3/If Action Subsystem1 ==
  In1 : Inport
  Action Port : ActionPort  ActionPortLabel=else
  Constant14 : Constant  Value=-2*pi
  Mod13 : Math  Operator=mod  SaturateOnIntegerOverflow=on
  Out1 : Outport
  wires:
  In1/1 -> Mod13/1
  Constant14/1 -> Mod13/2
  Mod13/1 -> Out1/1

== system blockdiagram/If Action Subsystem7/If Action Subsystem1/Subsystem7/If Action Subsystem3/If Action Subsystem3 ==
  In1 : Inport
  Action Port : ActionPort  InitializeStates=reset  ActionPortLabel=if(u1 >-ep)
  Out1 : Outport
  wires:
  In1/1 -> Out1/1

== system blockdiagram/If Action Subsystem7/If Action Subsystem7/If Action Subsystem1/Subsystem7/If Action Subsystem1 ==
  In1 : Inport
  Action Port : ActionPort  ActionPortLabel=else
  If Action Subsystem2 : Subsystem  TreatAsAtomicUnit=on
  If Action Subsystem4 : Subsystem  TreatAsAtomicUnit=on
  If1 : If  IfExpression=u1 <ep
  Merge1 : Merge
  Out1 : Outport
  wires:
  If1/1 -> If Action Subsystem4/Action
  If1/2 -> If Action Subsystem2/Action
  Merge1/1 -> Out1/1
  If Action Subsystem4/1(Out1) -> Merge1/1
  If Action Subsystem2/1(Out1) -> Merge1/2
  In1/1 -> If Action Subsystem2/1(In1), If Action Subsystem4/1(In1), If1/1

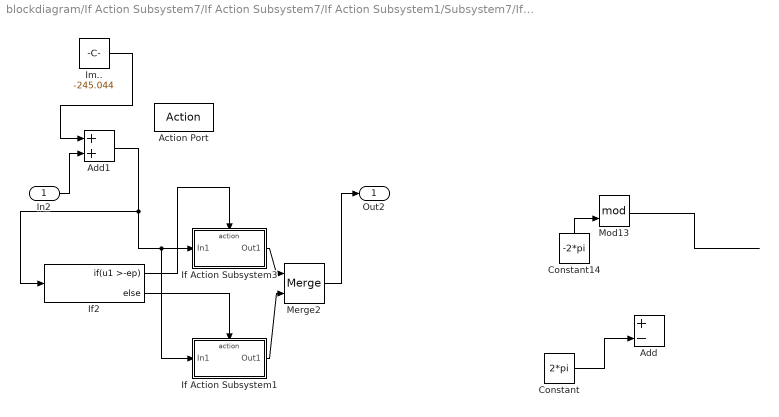
== system blockdiagram/If Action Subsystem7/If Action Subsystem7/If Action Subsystem1/Subsystem7/If Action Subsystem3 ==
  In2 : Inport
  Action Port : ActionPort  InitializeStates=reset  ActionPortLabel=if(u1 < 0)
  Add : Sum  Inputs=+-
  Add1 : Sum
  Constant : Constant  Value=2*pi
  Constant14 : Constant  Value=-2*pi
  If Action Subsystem1 : Subsystem  TreatAsAtomicUnit=on
  If Action Subsystem3 : Subsystem  TreatAsAtomicUnit=on
  If2 : If  IfExpression=u1 >-ep
  Im.. : Constant  Value=-245.044
  Merge2 : Merge
  Mod13 : Math  Operator=mod  SaturateOnIntegerOverflow=on
  Out2 : Outport
  wires:
  Mod13/1 -> ?
  Constant14/1 -> Mod13/2
  ? -> Mod13/1
  Constant/1 -> Add/2
  If Action Subsystem3/1(Out1) -> Merge2/1
  If2/1 -> If Action Subsystem3/Action
  If Action Subsystem1/1(Out1) -> Merge2/2
  If2/2 -> If Action Subsystem1/Action
  Merge2/1 -> Out2/1
  Im../1 -> Add1/1
  In2/1 -> Add1/2
  Add1/1 -> If Action Subsystem3/1(In1), If Action Subsystem1/1(In1), If2/1

== system blockdiagram/If Action Subsystem7/If Action Subsystem7/If Action Subsystem7/If Action Subsystem1/Subsystem7 ==
  In1 : Inport
  Derivative1 : Derivative
  If Action Subsystem1 : Subsystem  TreatAsAtomicUnit=on
  If Action Subsystem3 : Subsystem  TreatAsAtomicUnit=on
  If2 : If  IfExpression=u1 < 0
  Merge2 : Merge
  Out1 : Outport
  wires:
  Derivative1/1 -> If2/1
  If2/2 -> If Action Subsystem1/Action
  If Action Subsystem1/1(Out1) -> Merge2/2
  If Action Subsystem3/1(Out2) -> Merge2/1
  If2/1 -> If Action Subsystem3/Action
  In1/1 -> If Action Subsystem3/1(In2), If Action Subsystem1/1(In1), Derivative1/1
  Merge2/1 -> Out1/1

== system blockdiagram/If Action Subsystem7/If Action Subsystem7/If Action Subsystem7/If Action Subsystem2/If Action Subsystem2 ==
  In1 : Inport
  Action Port : ActionPort  ActionPortLabel=else
  Constant14 : Constant  Value=2*pi
  Mod13 : Math  Operator=mod  SaturateOnIntegerOverflow=on
  Out1 : Outport
  wires:
  In1/1 -> Mod13/1
  Constant14/1 -> Mod13/2
  Mod13/1 -> Out1/1

== system blockdiagram/If Action Subsystem7/If Action Subsystem7/If Action Subsystem7/If Action Subsystem2/If Action Subsystem4 ==
  In1 : Inport
  Action Port : ActionPort  InitializeStates=reset  ActionPortLabel=if(u1 <ep)
  Out1 : Outport
  wires:
  In1/1 -> Out1/1

== system blockdiagram/If Action Subsystem7/If Action Subsystem7/If Action Subsystem7/If Action Subsystem7/Subsystem7 ==
  In1 : Inport
  Derivative1 : Derivative
  If Action Subsystem1 : Subsystem  TreatAsAtomicUnit=on
  If Action Subsystem3 : Subsystem  TreatAsAtomicUnit=on
  If2 : If  IfExpression=u1 < 0
  Merge2 : Merge
  Out1 : Outport
  wires:
  Derivative1/1 -> If2/1
  If2/2 -> If Action Subsystem1/Action
  If Action Subsystem1/1(Out1) -> Merge2/2
  If Action Subsystem3/1(Out2) -> Merge2/1
  If2/1 -> If Action Subsystem3/Action
  In1/1 -> If Action Subsystem3/1(In2), If Action Subsystem1/1(In1), Derivative1/1
  Merge2/1 -> Out1/1

== system blockdiagram/If Action Subsystem7/If Action Subsystem7/Subsystem7/If Action Subsystem1/If Action Subsystem2 ==
  In1 : Inport
  Action Port : ActionPort  ActionPortLabel=else
  Constant14 : Constant  Value=2*pi
  Mod13 : Math  Operator=mod  SaturateOnIntegerOverflow=on
  Out1 : Outport
  wires:
  In1/1 -> Mod13/1
  Constant14/1 -> Mod13/2
  Mod13/1 -> Out1/1

== system blockdiagram/If Action Subsystem7/If Action Subsystem7/Subsystem7/If Action Subsystem1/If Action Subsystem4 ==
  In1 : Inport
  Action Port : ActionPort  InitializeStates=reset  ActionPortLabel=if(u1 <ep)
  Out1 : Outport
  wires:
  In1/1 -> Out1/1

== system blockdiagram/If Action Subsystem7/If Action Subsystem7/Subsystem7/If Action Subsystem3/If Action Subsystem1 ==
  In1 : Inport
  Action Port : ActionPort  ActionPortLabel=else
  Constant14 : Constant  Value=-2*pi
  Mod13 : Math  Operator=mod  SaturateOnIntegerOverflow=on
  Out1 : Outport
  wires:
  In1/1 -> Mod13/1
  Constant14/1 -> Mod13/2
  Mod13/1 -> Out1/1

== system blockdiagram/If Action Subsystem7/If Action Subsystem7/Subsystem7/If Action Subsystem3/If Action Subsystem3 ==
  In1 : Inport
  Action Port : ActionPort  InitializeStates=reset  ActionPortLabel=if(u1 >-ep)
  Out1 : Outport
  wires:
  In1/1 -> Out1/1

== system blockdiagram/If Action Subsystem7/If Action Subsystem7/If Action Subsystem1/Subsystem7/If Action Subsystem1/If Action Subsystem2 ==
  In1 : Inport
  Action Port : ActionPort  ActionPortLabel=else
  Constant14 : Constant  Value=2*pi
  Mod13 : Math  Operator=mod  SaturateOnIntegerOverflow=on
  Out1 : Outport
  wires:
  In1/1 -> Mod13/1
  Constant14/1 -> Mod13/2
  Mod13/1 -> Out1/1

== system blockdiagram/If Action Subsystem7/If Action Subsystem7/If Action Subsystem1/Subsystem7/If Action Subsystem1/If Action Subsystem4 ==
  In1 : Inport
  Action Port : ActionPort  InitializeStates=reset  ActionPortLabel=if(u1 <ep)
  Out1 : Outport
  wires:
  In1/1 -> Out1/1

== system blockdiagram/If Action Subsystem7/If Action Subsystem7/If Action Subsystem1/Subsystem7/If Action Subsystem3/If Action Subsystem1 ==
  In1 : Inport
  Action Port : ActionPort  ActionPortLabel=else
  Constant14 : Constant  Value=-2*pi
  Mod13 : Math  Operator=mod  SaturateOnIntegerOverflow=on
  Out1 : Outport
  wires:
  In1/1 -> Mod13/1
  Constant14/1 -> Mod13/2
  Mod13/1 -> Out1/1

== system blockdiagram/If Action Subsystem7/If Action Subsystem7/If Action Subsystem1/Subsystem7/If Action Subsystem3/If Action Subsystem3 ==
  In1 : Inport
  Action Port : ActionPort  InitializeStates=reset  ActionPortLabel=if(u1 >-ep)
  Out1 : Outport
  wires:
  In1/1 -> Out1/1

== system blockdiagram/If Action Subsystem7/If Action Subsystem7/If Action Subsystem7/If Action Subsystem1/Subsystem7/If Action Subsystem1 ==
  In1 : Inport
  Action Port : ActionPort  ActionPortLabel=else
  If Action Subsystem2 : Subsystem  TreatAsAtomicUnit=on
  If Action Subsystem4 : Subsystem  TreatAsAtomicUnit=on
  If1 : If  IfExpression=u1 <ep
  Merge1 : Merge
  Out1 : Outport
  wires:
  If1/1 -> If Action Subsystem4/Action
  If1/2 -> If Action Subsystem2/Action
  Merge1/1 -> Out1/1
  If Action Subsystem4/1(Out1) -> Merge1/1
  If Action Subsystem2/1(Out1) -> Merge1/2
  In1/1 -> If Action Subsystem2/1(In1), If Action Subsystem4/1(In1), If1/1

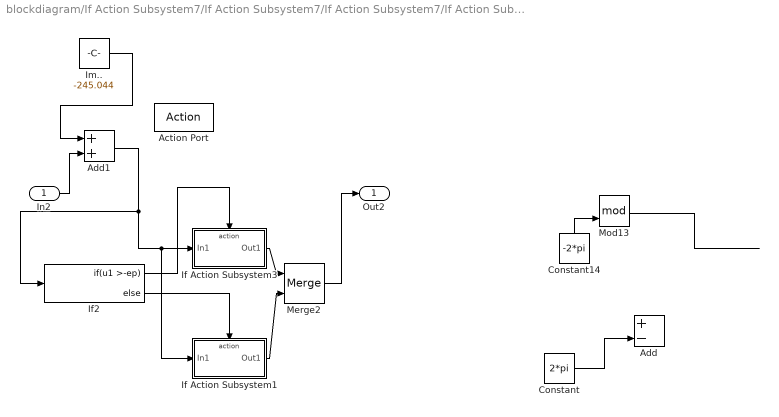
== system blockdiagram/If Action Subsystem7/If Action Subsystem7/If Action Subsystem7/If Action Subsystem1/Subsystem7/If Action Subsystem3 ==
  In2 : Inport
  Action Port : ActionPort  InitializeStates=reset  ActionPortLabel=if(u1 < 0)
  Add : Sum  Inputs=+-
  Add1 : Sum
  Constant : Constant  Value=2*pi
  Constant14 : Constant  Value=-2*pi
  If Action Subsystem1 : Subsystem  TreatAsAtomicUnit=on
  If Action Subsystem3 : Subsystem  TreatAsAtomicUnit=on
  If2 : If  IfExpression=u1 >-ep
  Im.. : Constant  Value=-245.044
  Merge2 : Merge
  Mod13 : Math  Operator=mod  SaturateOnIntegerOverflow=on
  Out2 : Outport
  wires:
  Mod13/1 -> ?
  Constant14/1 -> Mod13/2
  ? -> Mod13/1
  Constant/1 -> Add/2
  If Action Subsystem3/1(Out1) -> Merge2/1
  If2/1 -> If Action Subsystem3/Action
  If Action Subsystem1/1(Out1) -> Merge2/2
  If2/2 -> If Action Subsystem1/Action
  Merge2/1 -> Out2/1
  Im../1 -> Add1/1
  In2/1 -> Add1/2
  Add1/1 -> If Action Subsystem3/1(In1), If Action Subsystem1/1(In1), If2/1

== system blockdiagram/If Action Subsystem7/If Action Subsystem7/If Action Subsystem7/If Action Subsystem7/Subsystem7/If Action Subsystem1 ==
  In1 : Inport
  Action Port : ActionPort  ActionPortLabel=else
  If Action Subsystem2 : Subsystem  TreatAsAtomicUnit=on
  If Action Subsystem4 : Subsystem  TreatAsAtomicUnit=on
  If1 : If  IfExpression=u1 <ep
  Merge1 : Merge
  Out1 : Outport
  wires:
  If1/1 -> If Action Subsystem4/Action
  If1/2 -> If Action Subsystem2/Action
  Merge1/1 -> Out1/1
  If Action Subsystem4/1(Out1) -> Merge1/1
  If Action Subsystem2/1(Out1) -> Merge1/2
  In1/1 -> If Action Subsystem2/1(In1), If Action Subsystem4/1(In1), If1/1

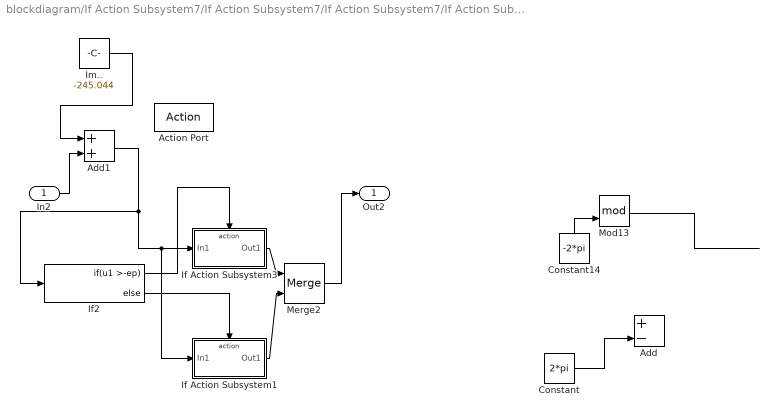
== system blockdiagram/If Action Subsystem7/If Action Subsystem7/If Action Subsystem7/If Action Subsystem7/Subsystem7/If Action Subsystem3 ==
  In2 : Inport
  Action Port : ActionPort  InitializeStates=reset  ActionPortLabel=if(u1 < 0)
  Add : Sum  Inputs=+-
  Add1 : Sum
  Constant : Constant  Value=2*pi
  Constant14 : Constant  Value=-2*pi
  If Action Subsystem1 : Subsystem  TreatAsAtomicUnit=on
  If Action Subsystem3 : Subsystem  TreatAsAtomicUnit=on
  If2 : If  IfExpression=u1 >-ep
  Im.. : Constant  Value=-245.044
  Merge2 : Merge
  Mod13 : Math  Operator=mod  SaturateOnIntegerOverflow=on
  Out2 : Outport
  wires:
  Mod13/1 -> ?
  Constant14/1 -> Mod13/2
  ? -> Mod13/1
  Constant/1 -> Add/2
  If Action Subsystem3/1(Out1) -> Merge2/1
  If2/1 -> If Action Subsystem3/Action
  If Action Subsystem1/1(Out1) -> Merge2/2
  If2/2 -> If Action Subsystem1/Action
  Merge2/1 -> Out2/1
  Im../1 -> Add1/1
  In2/1 -> Add1/2
  Add1/1 -> If Action Subsystem3/1(In1), If Action Subsystem1/1(In1), If2/1

== system blockdiagram/If Action Subsystem7/If Action Subsystem7/If Action Subsystem7/If Action Subsystem1/Subsystem7/If Action Subsystem1/If Action Subsystem2 ==
  In1 : Inport
  Action Port : ActionPort  ActionPortLabel=else
  Constant14 : Constant  Value=2*pi
  Mod13 : Math  Operator=mod  SaturateOnIntegerOverflow=on
  Out1 : Outport
  wires:
  In1/1 -> Mod13/1
  Constant14/1 -> Mod13/2
  Mod13/1 -> Out1/1

== system blockdiagram/If Action Subsystem7/If Action Subsystem7/If Action Subsystem7/If Action Subsystem1/Subsystem7/If Action Subsystem1/If Action Subsystem4 ==
  In1 : Inport
  Action Port : ActionPort  InitializeStates=reset  ActionPortLabel=if(u1 <ep)
  Out1 : Outport
  wires:
  In1/1 -> Out1/1

== system blockdiagram/If Action Subsystem7/If Action Subsystem7/If Action Subsystem7/If Action Subsystem1/Subsystem7/If Action Subsystem3/If Action Subsystem1 ==
  In1 : Inport
  Action Port : ActionPort  ActionPortLabel=else
  Constant14 : Constant  Value=-2*pi
  Mod13 : Math  Operator=mod  SaturateOnIntegerOverflow=on
  Out1 : Outport
  wires:
  In1/1 -> Mod13/1
  Constant14/1 -> Mod13/2
  Mod13/1 -> Out1/1

== system blockdiagram/If Action Subsystem7/If Action Subsystem7/If Action Subsystem7/If Action Subsystem1/Subsystem7/If Action Subsystem3/If Action Subsystem3 ==
  In1 : Inport
  Action Port : ActionPort  InitializeStates=reset  ActionPortLabel=if(u1 >-ep)
  Out1 : Outport
  wires:
  In1/1 -> Out1/1

== system blockdiagram/If Action Subsystem7/If Action Subsystem7/If Action Subsystem7/If Action Subsystem7/Subsystem7/If Action Subsystem1/If Action Subsystem2 ==
  In1 : Inport
  Action Port : ActionPort  ActionPortLabel=else
  Constant14 : Constant  Value=2*pi
  Mod13 : Math  Operator=mod  SaturateOnIntegerOverflow=on
  Out1 : Outport
  wires:
  In1/1 -> Mod13/1
  Constant14/1 -> Mod13/2
  Mod13/1 -> Out1/1

== system blockdiagram/If Action Subsystem7/If Action Subsystem7/If Action Subsystem7/If Action Subsystem7/Subsystem7/If Action Subsystem1/If Action Subsystem4 ==
  In1 : Inport
  Action Port : ActionPort  InitializeStates=reset  ActionPortLabel=if(u1 <ep)
  Out1 : Outport
  wires:
  In1/1 -> Out1/1

== system blockdiagram/If Action Subsystem7/If Action Subsystem7/If Action Subsystem7/If Action Subsystem7/Subsystem7/If Action Subsystem3/If Action Subsystem1 ==
  In1 : Inport
  Action Port : ActionPort  ActionPortLabel=else
  Constant14 : Constant  Value=-2*pi
  Mod13 : Math  Operator=mod  SaturateOnIntegerOverflow=on
  Out1 : Outport
  wires:
  In1/1 -> Mod13/1
  Constant14/1 -> Mod13/2
  Mod13/1 -> Out1/1

== system blockdiagram/If Action Subsystem7/If Action Subsystem7/If Action Subsystem7/If Action Subsystem7/Subsystem7/If Action Subsystem3/If Action Subsystem3 ==
  In1 : Inport
  Action Port : ActionPort  InitializeStates=reset  ActionPortLabel=if(u1 >-ep)
  Out1 : Outport
  wires:
  In1/1 -> Out1/1
